simulink model "stateobsrv"  (R2015a)
settings: Solver=ode45  StartTime=0.0  StopTime=10.0  RelTol=1e-3
values from neighbouring files (symbols this model uses):
  L = lqe(A, G, C, Qe, Re)    [L7.m]
undefined symbols (not defined in the file or in its folder): A, B, C, D, K, LC, x0
settings Model: Creator=afons  LastModifiedBy=afons

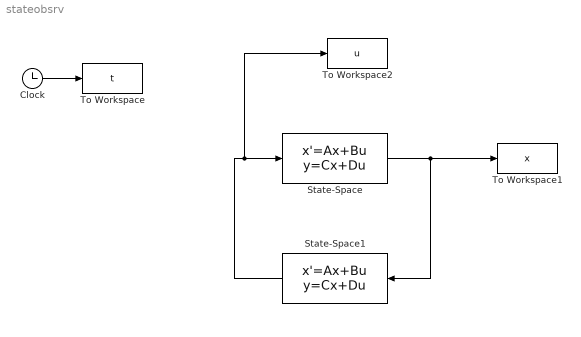
== system stateobsrv ==
  Clock : Clock
  State-Space : StateSpace  A=A  B=B  C=C  D=D  X0=x0
  State-Space1 : StateSpace  A=A -B*K -LC  B=L  C=-K  D=D  X0=x0
  To Workspace : ToWorkspace  VariableName=t  SaveFormat=Timeseries  SampleTime=-1
  To Workspace1 : ToWorkspace  VariableName=x  SaveFormat=Timeseries  SampleTime=-1
  To Workspace2 : ToWorkspace  VariableName=u  SaveFormat=Timeseries  SampleTime=-1
  wires:
  State-Space/1 -> State-Space1/1, To Workspace1/1
  Clock/1 -> To Workspace/1
  State-Space1/1 -> To Workspace2/1, State-Space/1
